simulink model "Nonlinear"  (R2021a)
settings: Solver=VariableStepAuto  StartTime=0.0  StopTime=10.0  MaxStep=0.1  RelTol=1
settings Model: Creator=mluser  LastModifiedBy=mluser
settings SolverCC: InitialStep=0.1

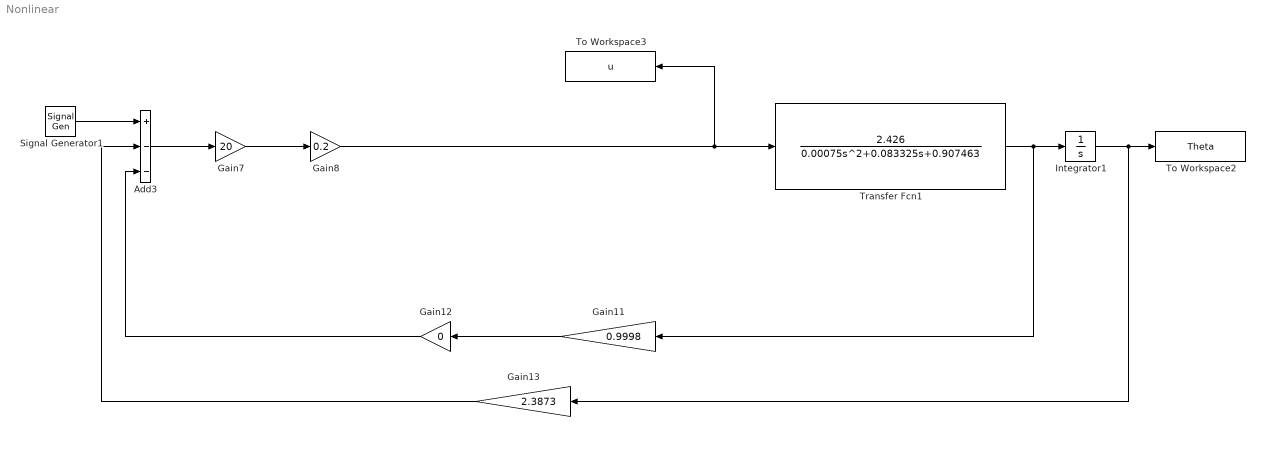
== system Nonlinear ==
  Add3 : Sum  Inputs=+--
  Gain11 : Gain  Gain=0.9998
  Gain12 : Gain  Gain=0
  Gain13 : Gain  Gain=2.3873
  Gain7 : Gain  Gain=20
  Gain8 : Gain  Gain=0.2
  Integrator1 : Integrator
  Signal Generator1 : SignalGenerator  WaveForm=square  Amplitude=2  Frequency=0.1
  To Workspace2 : ToWorkspace  VariableName=Theta  SaveFormat=Timeseries  SampleTime=-1
  To Workspace3 : ToWorkspace  VariableName=u  SaveFormat=Timeseries  SampleTime=-1
  Transfer Fcn1 : TransferFcn  Numerator=[2.426]  Denominator=[0.00075 0.083325 0.907463]
  wires:
  Add3/1 -> Gain7/1
  Integrator1/1 -> Gain13/1, To Workspace2/1
  Gain7/1 -> Gain8/1
  Signal Generator1/1 -> Add3/1
  Gain13/1 -> Add3/2
  Gain11/1 -> Gain12/1
  Gain12/1 -> Add3/3
  Transfer Fcn1/1 -> Gain11/1, Integrator1/1
  Gain8/1 -> To Workspace3/1, Transfer Fcn1/1
